simulink model "ASMC_test"  (R2021a)
settings: Solver=VariableStepAuto  StartTime=0.0  StopTime=10.0  RelTol=1e-3
settings Model: Creator=Zicx  LastModifiedBy=Zicx

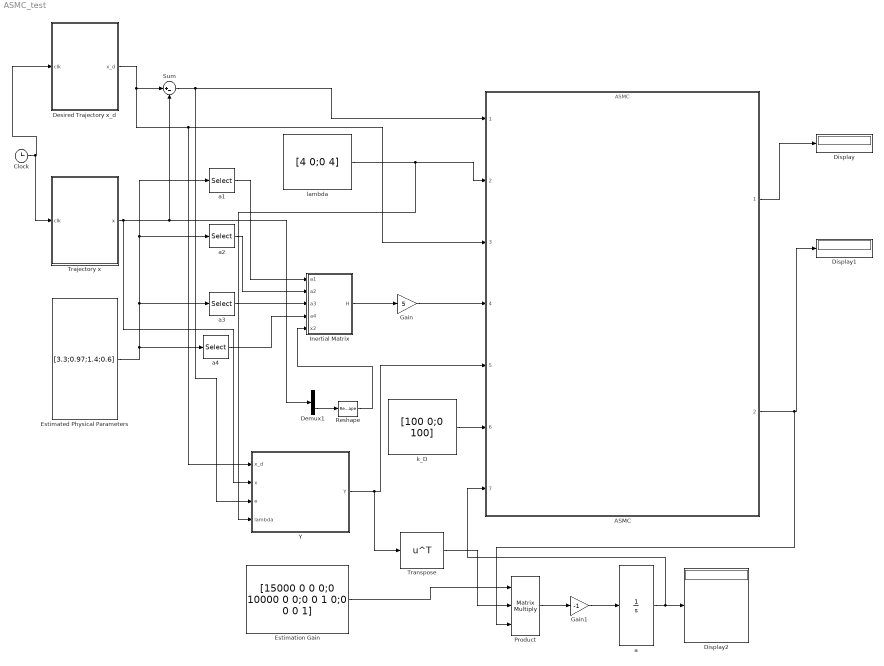
== system ASMC_test ==
  ASMC : ModelReference  ModelNameDialog=ASMC  SimulationMode=Normal  ModelReferenceVersion=1.84
  Clock : Clock
  Demux1 : Demux  Outputs=2
  Desired Trajectory x_d : Subsystem
  Display : Display
  Display1 : Display
  Display2 : Display
  Estimated Physical Parameters : Constant  Value=[3.3;0.97;1.4;0.6]
  Estimation Gain : Constant  Value=[15000 0 0 0;0 10000 0 0;0 0 1 0;0 0 0 1]
  Gain : Gain  Gain=5
  Gain1 : Gain  Gain=-1
  Inertial Matrix : Subsystem
  Product : Product  Inputs=3  Multiplication=Matrix(*)
  Reshape : Reshape  OutputDimensionality=Customize  OutputDimensions=1
  Sum : Sum  Inputs=|+-
  Trajectory x : Subsystem
  Transpose : Math  Operator=transpose  SaturateOnIntegerOverflow=on
  Y : Subsystem
  a : Integrator
  a1 : Selector  InputPortWidth=4  IndexOptions=Index vector (dialog)  Indices=[1]  OutputSizes=1
  a2 : Selector  InputPortWidth=4  IndexOptions=Index vector (dialog)  Indices=[2]  OutputSizes=1
  a3 : Selector  InputPortWidth=4  IndexOptions=Index vector (dialog)  Indices=[3]  OutputSizes=1
  a4 : Selector  InputPortWidth=4  IndexOptions=Index vector (dialog)  Indices=[4]  OutputSizes=1
  k_D : Constant  Value=[100 0;0 100]
  lambda : Constant  Value=[4 0;0 4]
  wires:
  Desired Trajectory x_d/1(x_d) -> Y/1(x_d), ASMC/3, Sum/1
  Clock/1 -> Trajectory x/1(clk), Desired Trajectory x_d/1(clk)
  Sum/1 -> Y/3(e), ASMC/1
  ASMC/1 -> Display/1
  ASMC/2 -> Product/3, Display1/1
  lambda/1 -> Y/4(lambda), ASMC/2
  a2/1 -> Inertial Matrix/2(a2)
  a1/1 -> Inertial Matrix/1(a1)
  Estimated Physical Parameters/1 -> a1/1, a2/1, a3/1, a4/1
  a3/1 -> Inertial Matrix/3(a3)
  a4/1 -> Inertial Matrix/4(a4)
  Trajectory x/1(x) -> Y/2(x), Demux1/1, Sum/2
  Demux1/2 -> Reshape/1
  Inertial Matrix/1(H) -> Gain/1
  Gain/1 -> ASMC/4
  Reshape/1 -> Inertial Matrix/5(x2)
  k_D/1 -> ASMC/6
  Gain1/1 -> a/1
  Product/1 -> Gain1/1
  a/1 -> ASMC/7, Display2/1
  Estimation Gain/1 -> Product/1
  Y/1(Y) -> ASMC/5, Transpose/1
  Transpose/1 -> Product/2

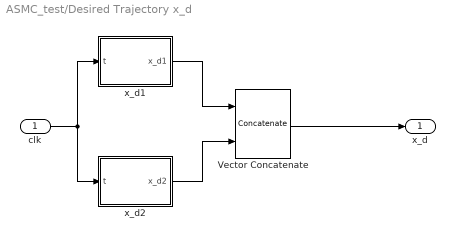
== system ASMC_test/Desired Trajectory x_d ==
  clk : Inport
  Vector Concatenate : Concatenate
  x_d1 : MATLAB Function  TreatAsAtomicUnit=on
  x_d2 : MATLAB Function  TreatAsAtomicUnit=on
  x_d : Outport
  wires:
  clk/1 -> x_d2/1(t), x_d1/1(t)
  x_d1/1(x_d1) -> Vector Concatenate/1
  Vector Concatenate/1 -> x_d/1
  x_d2/1(x_d2) -> Vector Concatenate/2

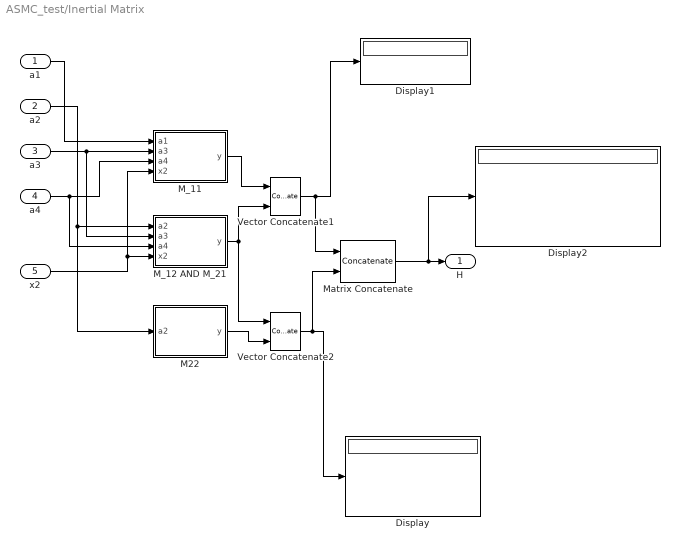
== system ASMC_test/Inertial Matrix ==
  a1 : Inport
  a2 : Inport  Port=2
  a3 : Inport  Port=3
  a4 : Inport  Port=4
  x2 : Inport  Port=5
  Display : Display
  Display1 : Display
  Display2 : Display
  M22 : MATLAB Function  TreatAsAtomicUnit=on
  M_11 : MATLAB Function  TreatAsAtomicUnit=on
  M_12 AND M_21 : MATLAB Function  TreatAsAtomicUnit=on
  Matrix Concatenate : Concatenate  Mode=Multidimensional array  ConcatenateDimension=2
  Vector Concatenate1 : Concatenate
  Vector Concatenate2 : Concatenate
  H : Outport
  wires:
  Matrix Concatenate/1 -> Display2/1, H/1
  a1/1 -> M_11/1(a1)
  a3/1 -> M_11/2(a3), M_12 AND M_21/2(a3)
  a4/1 -> M_11/3(a4), M_12 AND M_21/3(a4)
  a2/1 -> M22/1(a2), M_12 AND M_21/1(a2)
  Vector Concatenate2/1 -> Display/1, Matrix Concatenate/2
  M22/1(y) -> Vector Concatenate2/2
  Vector Concatenate1/1 -> Display1/1, Matrix Concatenate/1
  M_12 AND M_21/1(y) -> Vector Concatenate2/1, Vector Concatenate1/2
  x2/1 -> M_12 AND M_21/4(x2), M_11/4(x2)
  M_11/1(y) -> Vector Concatenate1/1

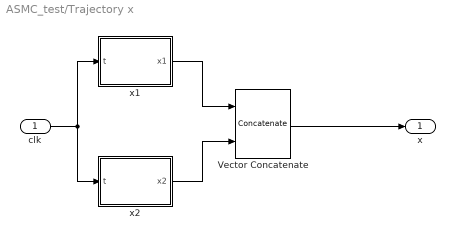
== system ASMC_test/Trajectory x ==
  clk : Inport
  Vector Concatenate : Concatenate
  x1 : MATLAB Function  TreatAsAtomicUnit=on
  x2 : MATLAB Function  TreatAsAtomicUnit=on
  x : Outport
  wires:
  clk/1 -> x2/1(t), x1/1(t)
  x1/1(x1) -> Vector Concatenate/1
  Vector Concatenate/1 -> x/1
  x2/1(x2) -> Vector Concatenate/2

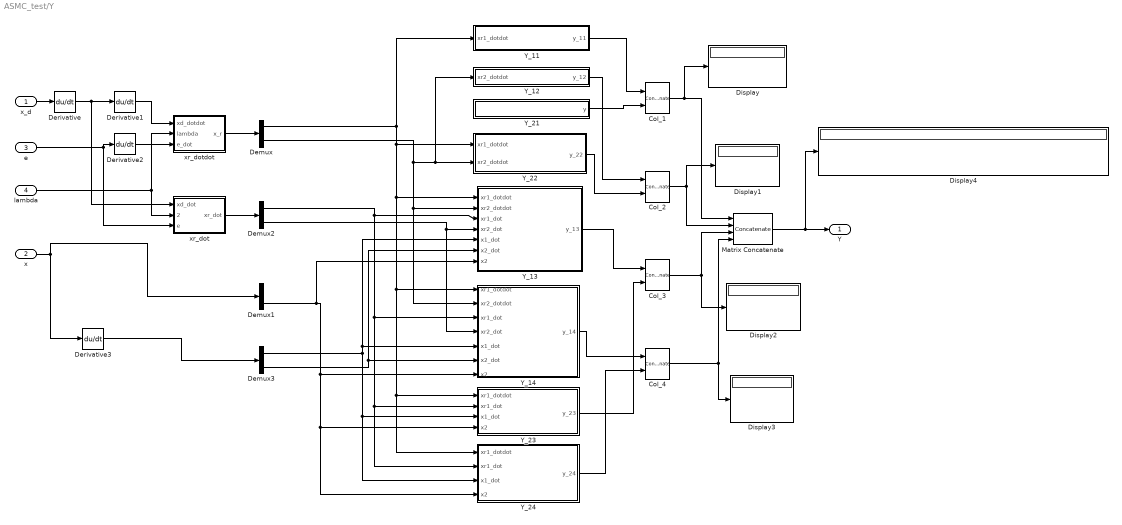
== system ASMC_test/Y ==
  x_d : Inport
  x : Inport  Port=2
  e : Inport  Port=3
  lambda : Inport  Port=4
  Col_{1..4} (4 alike) : Concatenate
  Demux{,1..3} (4 alike) : Demux  Outputs=2
  Derivative{,1..3} (4 alike) : Derivative
  Display{,1..4} (5 alike) : Display
  Matrix Concatenate : Concatenate  NumInputs=4  Mode=Multidimensional array  ConcatenateDimension=2
  Y_11 : MATLAB Function  TreatAsAtomicUnit=on
  Y_12 : MATLAB Function  TreatAsAtomicUnit=on
  Y_13 : MATLAB Function  TreatAsAtomicUnit=on
  Y_14 : MATLAB Function  TreatAsAtomicUnit=on
  Y_21 : MATLAB Function  TreatAsAtomicUnit=on
  Y_22 : MATLAB Function  TreatAsAtomicUnit=on
  Y_23 : MATLAB Function  TreatAsAtomicUnit=on
  Y_24 : MATLAB Function  TreatAsAtomicUnit=on
  xr_dot : MATLAB Function  TreatAsAtomicUnit=on
  xr_dotdot : MATLAB Function  TreatAsAtomicUnit=on
  Y : Outport
  wires:
  Demux3/2 -> Y_13/6(x2_dot), Y_14/6(x2_dot)
  Demux2/2 -> Y_13/4(xr2_dot), Y_14/4(xr2_dot)
  Y_14/1(y_14) -> Col_4/1
  Demux1/2 -> Y_13/7(x2), Y_14/7(x2), Y_23/4(x2), Y_24/4(x2)
  Col_1/1 -> Display/1, Matrix Concatenate/1
  Y_21/1(y) -> Col_1/2
  Demux2/1 -> Y_13/3(xr1_dot), Y_14/3(xr1_dot), Y_23/2(xr1_dot), Y_24/2(xr1_dot)
  e/1 -> xr_dot/3(e), Derivative2/1
  lambda/1 -> xr_dotdot/2(lambda), xr_dot/2(lambda)
  Y_12/1(y_12) -> Col_2/1
  Y_11/1(y_11) -> Col_1/1
  Derivative3/1 -> Demux3/1
  Y_24/1(y_24) -> Col_4/2
  Col_2/1 -> Display1/1, Matrix Concatenate/2
  Demux3/1 -> Y_24/3(x1_dot), Y_23/3(x1_dot), Y_14/5(x1_dot), Y_13/5(x1_dot)
  x_d/1 -> Derivative/1
  Y_22/1(y_22) -> Col_2/2
  Derivative/1 -> xr_dot/1(xd_dot), Derivative1/1
  Y_23/1(y_23) -> Col_3/2
  Matrix Concatenate/1 -> Display4/1, Y/1
  xr_dot/1(xr_dot) -> Demux2/1
  Col_4/1 -> Matrix Concatenate/4, Display3/1
  xr_dotdot/1(x_r) -> Demux/1
  x/1 -> Demux1/1, Derivative3/1
  Derivative1/1 -> xr_dotdot/1(xd_dotdot)
  Demux/1 -> Y_13/1(xr1_dotdot), Y_23/1(xr1_dotdot), Y_24/1(xr1_dotdot), Y_14/1(xr1_dotdot), Y_22/1(xr1_dotdot), Y_11/1(xr1_dotdot)
  Y_13/1(y_13) -> Col_3/1
  Col_3/1 -> Display2/1, Matrix Concatenate/3
  Derivative2/1 -> xr_dotdot/3(e_dot)
  Demux/2 -> Y_14/2(xr2_dotdot), Y_13/2(xr2_dotdot), Y_12/1(xr2_dotdot), Y_22/2(xr2_dotdot)

== matlab function ASMC_test/Y/Y_23 ==
  data: xr1_dotdot input; y_23 output; xr1_dot input; x1_dot input; x2 input
function y_23 = fcn(xr1_dotdot, xr1_dot, x1_dot, x2)

y_23 = xr1_dotdot * cos(x2) + x1_dot * xr1_dot * sin(x2);

== matlab function ASMC_test/Y/Y_24 ==
  data: xr1_dotdot input; y_24 output; xr1_dot input; x1_dot input; x2 input
function y_24 = fcn(xr1_dotdot, xr1_dot, x1_dot, x2)

y_24 = xr1_dotdot * sin(x2) - x1_dot * xr1_dot * cos(x2);

== matlab function ASMC_test/Y/xr_dotdot ==
  data: xd_dotdot input; x_r output; lambda input; e_dot input
function x_r = fcn(xd_dotdot, lambda, e_dot)

x_r = xd_dotdot - lambda * e_dot;

== matlab function ASMC_test/Desired Trajectory x_d/x_d2 ==
  data: t input; x_d2 output
function x_d2 = fcn(t)

x_d2 = pi/6 * (1 - cos(2 * pi * t) + sin(1.5 * pi * t));

== matlab function ASMC_test/Y/xr_dot ==
  data: xd_dot input; xr_dot output; lambda input; e input
function xr_dot = fcn(xd_dot, lambda, e)

xr_dot = xd_dot - lambda * e;

== matlab function ASMC_test/Y/Y_14 ==
  data: xr1_dotdot input; y_14 output; xr2_dotdot input; xr1_dot input; xr2_dot input; x1_dot input; x2_dot input; x2 input
function y_14 = fcn(xr1_dotdot, xr2_dotdot, xr1_dot, xr2_dot, x1_dot, x2_dot, x2)

y_14 = (2*xr1_dotdot+xr2_dotdot)*sin(x2) + (x2_dot*xr1_dot + x1_dot*xr2_dot + x2_dot*xr2_dot)*cos(x2);

== matlab function ASMC_test/Desired Trajectory x_d/x_d1 ==
  data: t input; x_d1 output
function x_d1 = fcn(t)

x_d1 = pi/6 * (1 - cos(1.5 * pi * t) + sin(pi * t));

== matlab function ASMC_test/Trajectory x/x1 ==
  data: t input; x1 output
function x1 = fcn(t)

x1 = pi/3 * (1 - cos(1.5 * pi * t));

== matlab function ASMC_test/Trajectory x/x2 ==
  data: t input; x2 output
function x2 = fcn(t)

x2 = pi/6 * sin(1.5 * pi * t);

== matlab function ASMC_test/Y/Y_11 ==
  data: xr1_dotdot input; y_11 output
function y_11 = fcn(xr1_dotdot)

y_11 = xr1_dotdot;

== matlab function ASMC_test/Inertial Matrix/M22 ==
  data: a2 input; y output
function y = fcn(a2)

y = a2;

== matlab function ASMC_test/Inertial Matrix/M_11 ==
  data: a1 input; a3 input; a4 input; y output; x2 input
function y = fcn(a1, a3, a4, x2)
%#codegen

y = a1 + 2*a3 * cos(x2)- 2 * a4 * sin(x2);

== matlab function ASMC_test/Inertial Matrix/M_12 AND M_21 ==
  data: a2 input; y output; a3 input; a4 input; x2 input
function y = fcn(a2, a3, a4, x2)

y = a2 + a3 * cos(x2) + a4 * sin(x2);

== matlab function ASMC_test/Y/Y_12 ==
  data: xr2_dotdot input; y_12 output
function y_12 = fcn(xr2_dotdot)

y_12 = xr2_dotdot;

== matlab function ASMC_test/Y/Y_21 ==
  data: y output
function y = fcn()

y = 0;

== matlab function ASMC_test/Y/Y_22 ==
  data: xr1_dotdot input; y_22 output; xr2_dotdot input
function y_22 = fcn(xr1_dotdot, xr2_dotdot)

y_22 = xr1_dotdot + xr2_dotdot;

== matlab function ASMC_test/Y/Y_13 ==
  data: xr1_dotdot input; y_13 output; xr2_dotdot input; xr1_dot input; xr2_dot input; x1_dot input; x2_dot input; x2 input
function y_13 = fcn(xr1_dotdot, xr2_dotdot, xr1_dot, xr2_dot, x1_dot, x2_dot, x2)

y_13 = (2*xr1_dotdot+xr2_dotdot)*cos(x2) - (x2_dot*xr1_dot + x1_dot*xr2_dot + x2_dot*xr2_dot)*sin(x2);
